simulink model "linearLatDir"  (R2024b)
settings: Solver=VariableStepAuto  StartTime=0.0  StopTime=25  RelTol=1e-3
settings Model: Creator=pablo  LastModifiedBy=himma
settings SolverCC: AlgebraicLoopSolver=TrustRegion
settings DebuggingCC: UnconnectedInputMsg=warning  UnconnectedOutputMsg=warning  UnconnectedLineMsg=warning  ArithmeticOperatorsInVariantConditions=warning
settings ModelReferenceCC: EnableRefExpFcnMdlSchedulingChecks=on
settings SFSimCC: CustomCodeUndefinedFunction=UseInterfaceOnly
settings RTWCC: GPUComputeCapability=3.5  DLArmComputeVersion=19.05

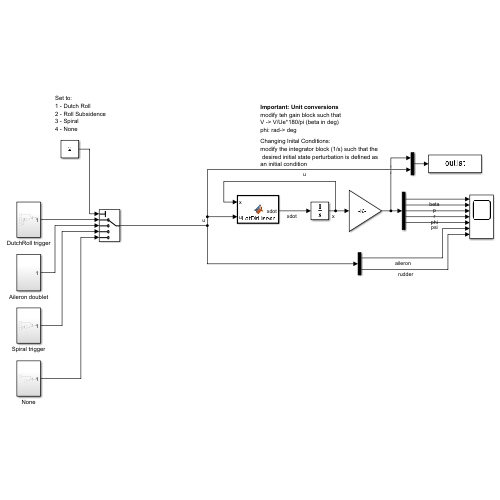
[thumbnail: Simulink's stored preview of the top-level diagram]
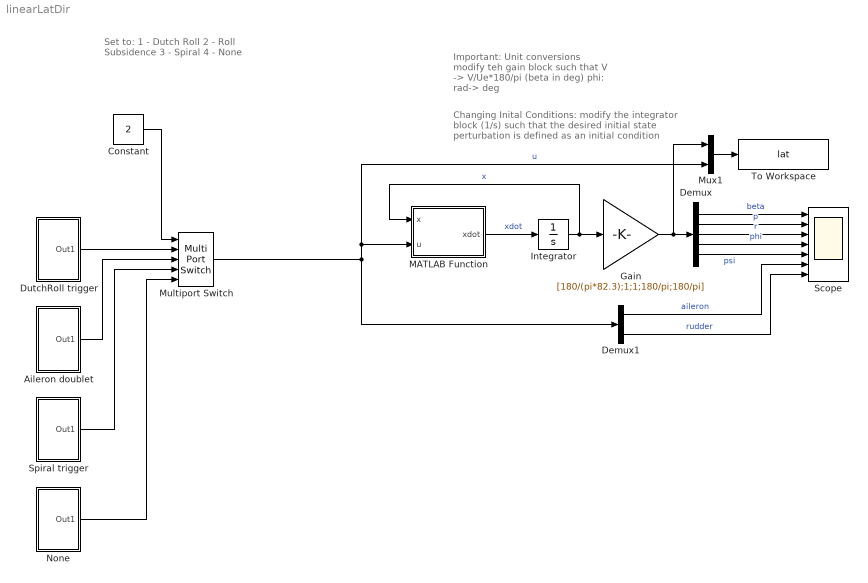
== system linearLatDir ==
  note: Set to:
      | 1 - Dutch Roll
      | 2 - Roll Subsidence
      | 3 - Spiral
      | 4 - None
  note: Important: Unit conversions
      | modify teh gain block such that
      | V -> V/Ue*180/pi (beta in deg)
      | phi: rad-> deg
  note: Changing Inital Conditions:
      | modify the integrator block (1/s) such that the
      | desired initial state perturbation is defined as
      | an initial condition
  Aileron doublet : Subsystem
  Constant : Constant  Value=2
  Demux : Demux  Outputs=5
  Demux1 : Demux  Outputs=2
  DutchRoll trigger : Subsystem
  Gain : Gain  Gain=[180/(pi*82.3);1;1;180/pi;180/pi]
  Integrator : Integrator  InitialCondition=[0;0;0;0;0]
  MATLAB Function : MATLAB Function  TreatAsAtomicUnit=on
  Multiport Switch : MultiPortSwitch  Inputs=4  SaturateOnIntegerOverflow=off  InputSameDT=off
  Mux1 : Mux  Inputs=2
  None : Subsystem
  Scope : Scope  NumInputPorts=7
  Spiral trigger : Subsystem
  To Workspace : ToWorkspace  VariableName=lat  SaveFormat=Timeseries  SampleTime=0.01
  wires:
  MATLAB Function/1(xdot) -> Integrator/1  "xdot"
  Integrator/1 -> MATLAB Function/1(x), Gain/1  "x"
  Gain/1 -> Mux1/1, Demux/1
  Demux/1 -> Scope/1  "beta"
  Demux/2 -> Scope/2  "p"
  Demux/3 -> Scope/3  "r"
  Demux/4 -> Scope/4  "phi"
  DutchRoll trigger/1(Out1) -> Multiport Switch/2
  Demux1/1 -> Scope/6  "aileron"
  Demux1/2 -> Scope/7  "rudder"
  Mux1/1 -> To Workspace/1
  Multiport Switch/1 -> MATLAB Function/2(u), Mux1/2, Demux1/1  "u"
  Aileron doublet/1(Out1) -> Multiport Switch/3
  Spiral trigger/1(Out1) -> Multiport Switch/4
  Constant/1 -> Multiport Switch/1
  Demux/5 -> Scope/5  "psi"
  None/1(Out1) -> Multiport Switch/5

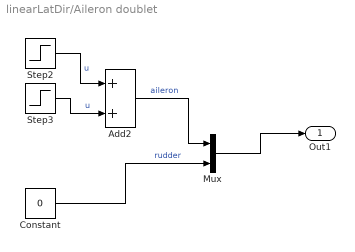
== system linearLatDir/Aileron doublet ==
  Add2 : Sum
  Constant : Constant  Value=0
  Mux : Mux  Inputs=2
  Step2 : Step  Time=0.8  SampleTime=0
  Step3 : Step  Time=1.6  After=-1  SampleTime=0
  Out1 : Outport  VectorParamsAs1DForOutWhenUnconnected=off
  wires:
  Mux/1 -> Out1/1
  Add2/1 -> Mux/1  "aileron"
  Step2/1 -> Add2/1  "u"
  Constant/1 -> Mux/2  "rudder"
  Step3/1 -> Add2/2  "u"

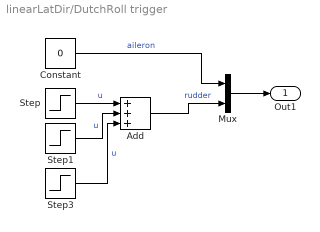
== system linearLatDir/DutchRoll trigger ==
  Add : Sum  Inputs=+++
  Constant : Constant  Value=0
  Mux : Mux  Inputs=2
  Step : Step  Time=0.6  SampleTime=0
  Step1 : Step  Time=1.2  After=-2  SampleTime=0
  Step3 : Step  Time=1.8  SampleTime=0
  Out1 : Outport
  wires:
  Add/1 -> Mux/2  "rudder"
  Step1/1 -> Add/2  "u"
  Step/1 -> Add/1  "u"
  Constant/1 -> Mux/1  "aileron"
  Mux/1 -> Out1/1
  Step3/1 -> Add/3  "u"

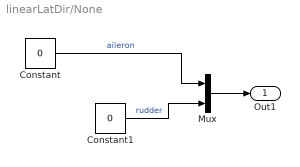
== system linearLatDir/None ==
  Constant : Constant  Value=0
  Constant1 : Constant  Value=0
  Mux : Mux  Inputs=2
  Out1 : Outport
  wires:
  Constant1/1 -> Mux/2  "rudder"
  Constant/1 -> Mux/1  "aileron"
  Mux/1 -> Out1/1

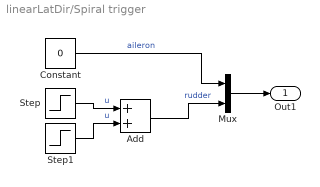
== system linearLatDir/Spiral trigger ==
  Add : Sum
  Constant : Constant  Value=0
  Mux : Mux  Inputs=2
  Step : Step  Time=0.6  SampleTime=0
  Step1 : Step  Time=1.2  After=-1  SampleTime=0
  Out1 : Outport
  wires:
  Add/1 -> Mux/2  "rudder"
  Step1/1 -> Add/2  "u"
  Step/1 -> Add/1  "u"
  Constant/1 -> Mux/1  "aileron"
  Mux/1 -> Out1/1

== matlab function linearLatDir/MATLAB Function ==
  data: x input; u input; xdot output
function xdot = LatDirLinear(x,u)
%inputs - x: (5x1)lateral state vector
%         x(1)- v   m/s
%         x(2)- p   rad/s
%         x(3)- r   rad/s
%         x(4)- phi rad
%         x(5)- psi rad
%       - u: lateral control vector
%         u(1)- aileron deflection as percentage
%         u(2)- rudder deflection as percentage
%Outputs-xdot:(5x1)
%Define parameters for aircraft
m = ; %kg
Ixx = ;%kg m^2
Izx = ;%kg m^2
Izz = ;%kg m^2
Ue = ;%m/s
g = 9.81; %m/s^2
theta = 0; %rad

Yv = ; %Ns/m
Yp = ; %Ns
Yr = ; %Ns
Lv = ; %Ns
Lp = ; %Nms
Lr = ; %Nms
Nv = ; %Ns
Np = ; %Nms
Nr = ; %Nms
%Aileron input
Y_a = ; 
L_a = ; %Rolling moment due to aileron deflection in RAD - Nm
N_a = ;
%Rudder input
Y_r = ; %Sideforce derivative with rudder in RAD - Nm
L_r = ; %Rolling moment derivative with rudder in RAD - Nm
N_r = ; %Yawing moment derivative with rudder in RAD - Nm

M = [
    

    ];

A = [
    


    ];

B = [
    


    ];

u=u.*[25,-30]*pi/180; %convert percentage to angle in rad
xdot = M\(A*x+B*u);
